simulink model "camera_radar_lidar"  (R2021b)
settings: Solver=FixedStepDiscrete  StartTime=0.0  StopTime=10.0  RelTol=1e-3
model workspace (MAT data in the model file):
  firstWarning = 1
  originalScenarioChecksum = 'D0B0A4B173DD3DA6100BB92ACC3E01B4'
undefined symbols (not defined in the file or in its folder): driving
libraries: drivingscenarioandsensors x7, sensorinslib x1
(part 2 of 22)

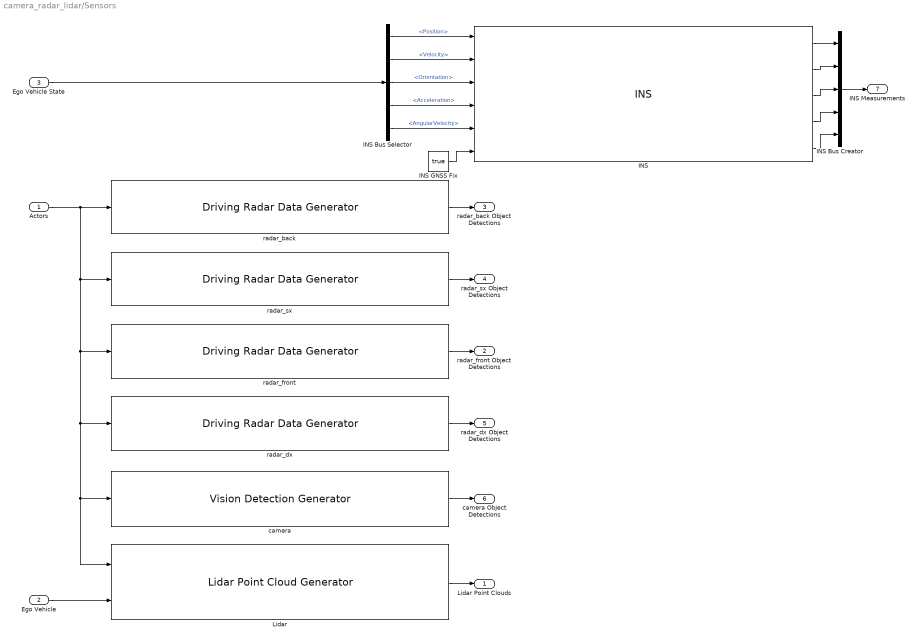
== system camera_radar_lidar/Sensors ==
  Actors : Inport
  Ego Vehicle : Inport  Port=2
  Ego Vehicle State : Inport  Port=3
  INS : sensorinslib/INS  MountingLocation=[0.05 0 0]  RollAccuracy=0.2  PitchAccuracy=0.2  YawAccuracy=1  PositionAccuracy=[1 1 1]  VelocityAccuracy=0.05  UseAccelAndAngVel=on  AccelerationAccuracy=0  AngularVelocityAccuracy=0  TimeInput=on  PositionErrorFactor=[0 0 0]  SeedDouble=67  SimulateUsing=Code generation
      settings: SourceProductBaseCode=DR,TF,NV,UV
  INS Bus Creator : BusCreator  Inputs=5
  INS Bus Selector : BusSelector  OutputSignals=Position,Velocity,Orientation,Acceleration,AngularVelocity
  INS GNSS Fix : Constant  Value=true
  Lidar : drivingscenarioandsensors/Lidar Point Cloud Generator  SensorIndex=1  UpdateInterval=0.1  SensorLocation=[0.05 0]  Height=1.6  Yaw=0  Pitch=0  Roll=0  DetectionCoordinates=Ego Cartesian  HasEgoVehicle=on  EgoVehicleActorID=2  HasRoadsInputPort=on  ActorProfilesSource=From Scenario Reader block  ActorProfilesVariableName=actor_profiles  MaxRange=50  RangeAccuracy=0.002  AzimuthResolution=0.16  ElevationResolution=1.25  AzimuthLimits=[-180 180]  ElevationLimits=[-20 20]  HasNoise=on
      settings: SourceProductBaseCode=DR
